simulink model "log2_fixed_point"  (R2018b)
settings: Solver=FixedStepDiscrete  StartTime=0.0  StopTime=1e6  RelTol=1e-3  EnableMultiTasking=on
InitFcn:
  | set_log2_fixed_point_params
undefined symbols (not defined in the file or in its folder): log2_fixed_point
libraries: hdlsllib x22, simulink x8
settings Model: FPTRunName=FPA_Reference  Creator=minimales  LastModifiedBy=ekorotkyi
settings OptimizationCC: BlockReduction=off  ConditionallyExecuteInputs=off  DefaultParameterBehavior=Inlined  LifeSpan=inf
settings DebuggingCC: AlgebraicLoopMsg=error  SingleTaskRateTransMsg=error  SFUnexpectedBacktrackingDiag=warning  SFNoUnconditionalDefaultTransitionDiag=warning  SFExecutionAtInitializationDiag=none
settings HardwareCC: ProdBitPerPointer=32  ProdBitPerSizeT=32  ProdBitPerPtrDiffT=32  ProdLargestAtomicFloat=None  ProdIntDivRoundTo=Undefined  ProdEndianess=Unspecified  ProdWordSize=32  ProdHWDeviceType=ASIC/FPGA->ASIC/FPGA  ProdEqTarget=off
settings SFSimCC: SimUseLocalCustomCode=off
settings RTWCC: RTWUseLocalCustomCode=off
settings CodeAppCC: StateflowObjectComments=on
settings GRTTargetCC: TargetLangStandard=C89/C90 (ANSI)  GeneratePreprocessorConditionals=Disable all
settings ConfigComp: CovScope=Subsystem  CovPath=SIGNAL_PROCESSING_DF  CovMetricSettings=w  CovHTMLOptions=-sRT=1 -sVT=0 -aTS=1 -bRG=1 -bTC=1 -hTR=0 -nFC=0 -nFD=1 -scm=1 -bcm=1 -xEv=0 -xEM=0  CovHtmlReporting=on  CovSaveCumulativeToWorkspaceVar=on  CovSaveSingleToWorkspaceVar=on  CovExternalEMLEnable=off  CovSFcnEnable=off

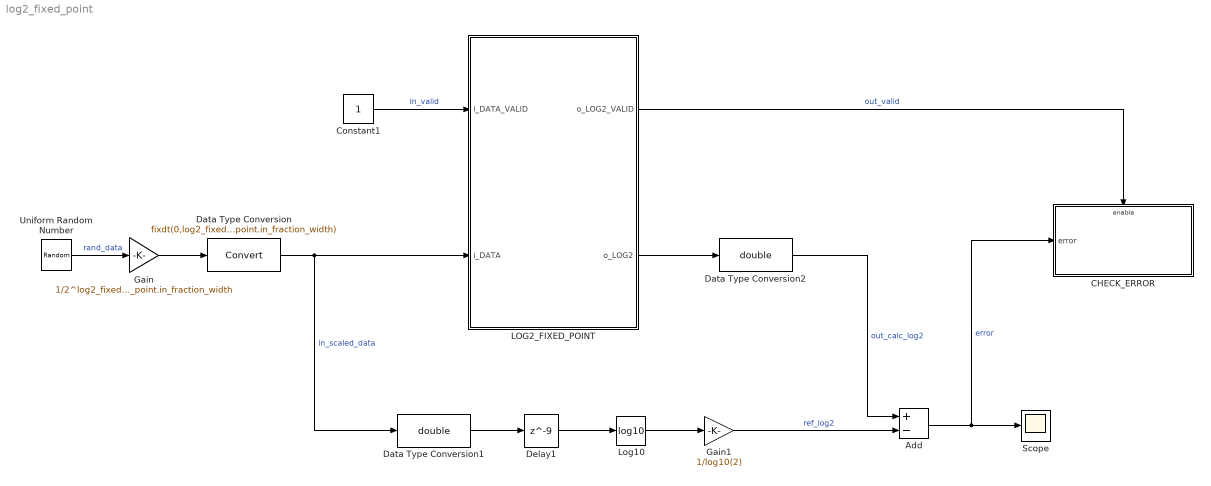
== system log2_fixed_point ==
  Add : Sum  Inputs=+-
  CHECK_ERROR : Subsystem
  Constant1 : Constant  OutDataTypeStr=boolean  SampleTime=1
  Data Type Conversion : DataTypeConversion  OutDataTypeStr=fixdt(0,log2_fixed_point.in_word_width,log2_fixed_point.in_fraction_width)
  Data Type Conversion1 : DataTypeConversion  OutDataTypeStr=double
  Data Type Conversion2 : DataTypeConversion  OutDataTypeStr=double
  Delay1 : Delay  DelayLength=9  InitialCondition=0
  Gain : Gain  Gain=1/2^log2_fixed_point.in_fraction_width
  Gain1 : Gain  Gain=1/log10(2)
  LOG2_FIXED_POINT : Subsystem
  Log10 : Math  Operator=log10  SaturateOnIntegerOverflow=on
  Scope : Scope
  Uniform Random Number : UniformRandomNumber  Minimum=2^(log2_fixed_point.in_word_width-1)  Maximum=2^log2_fixed_point.in_word_width-1  SampleTime=1
  wires:
  LOG2_FIXED_POINT/1(o_LOG2_VALID) -> CHECK_ERROR/Enable  "out_valid"
  LOG2_FIXED_POINT/2(o_LOG2) -> Data Type Conversion2/1
  Constant1/1 -> LOG2_FIXED_POINT/1(i_DATA_VALID)  "in_valid"
  Data Type Conversion/1 -> LOG2_FIXED_POINT/2(i_DATA), Data Type Conversion1/1  "in_scaled_data"
  Log10/1 -> Gain1/1
  Add/1 -> CHECK_ERROR/1(error), Scope/1  "error"
  Gain/1 -> Data Type Conversion/1
  Data Type Conversion2/1 -> Add/1  "out_calc_log2"
  Gain1/1 -> Add/2  "ref_log2"
  Delay1/1 -> Log10/1
  Uniform Random Number/1 -> Gain/1  "rand_data"
  Data Type Conversion1/1 -> Delay1/1

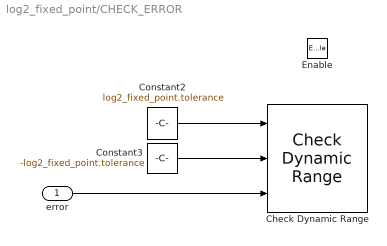
== system log2_fixed_point/CHECK_ERROR ==
  error : Inport
  Enable : EnablePort
  Check Dynamic Range : simulink/Model Verification/Check  Dynamic Range  Description=min < u < max  enabled=on  stopWhenAssertionFail=on  export=off  icon=graphic
      settings: SourceProductName=Simulink  SourceProductBaseCode=SL
  Constant2 : Constant  Value=log2_fixed_point.tolerance  OutDataTypeStr=double  SampleTime=1
  Constant3 : Constant  Value=-log2_fixed_point.tolerance  OutDataTypeStr=double  SampleTime=1
  wires:
  Constant3/1 -> Check Dynamic Range/2
  Constant2/1 -> Check Dynamic Range/1
  error/1 -> Check Dynamic Range/3

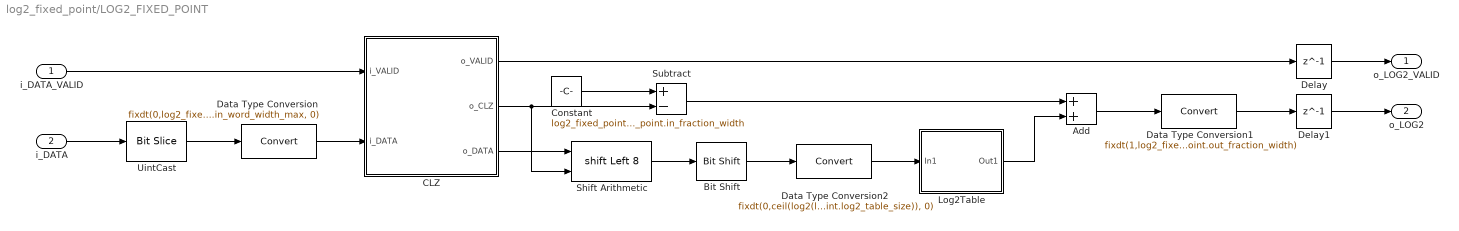
== system log2_fixed_point/LOG2_FIXED_POINT ==
  i_DATA_VALID : Inport  OutDataTypeStr=boolean
  i_DATA : Inport  Port=2  OutDataTypeStr=fixdt(0,log2_fixed_point.in_word_width,log2_fixed_point.in_fraction_width)
  Add : Sum
  Bit Shift : hdlsllib/Logic and Bit Operations/Bit Shift  mode=Shift Right Logical  N=log2_fixed_point.in_word_width_max- (ceil(log2(log2_fixed_point.log2_table_size))+1)
      settings: SourceProductName=HDL Coder  SourceProductBaseCode=HD
  CLZ : Subsystem
  Constant : Constant  Value=log2_fixed_point.in_word_width_max - 1 - log2_fixed_point.in_fraction_width  OutDataTypeStr=fixdt(0,ceil(log2(log2_fixed_point.in_word_width_max)) + 1,0)  SampleTime=1
  Data Type Conversion : DataTypeConversion  OutDataTypeStr=fixdt(0,log2_fixed_point.in_word_width_max, 0)
  Data Type Conversion1 : DataTypeConversion  OutDataTypeStr=fixdt(1,log2_fixed_point.out_word_width,log2_fixed_point.out_fraction_width)
  Data Type Conversion2 : DataTypeConversion  OutDataTypeStr=fixdt(0,ceil(log2(log2_fixed_point.log2_table_size)), 0)
  Delay : Delay  DelayLength=1  InitialCondition=0
  Delay1 : Delay  DelayLength=1  InitialCondition=0
  Log2Table : Subsystem
  Shift Arithmetic : ArithShift  BitShiftNumberSource=Input port  BitShiftNumber=8  BitShiftDirection=Left
      settings: InputPortMap=u0,p1
  Subtract : Sum  Inputs=+-
  UintCast : hdlsllib/Logic and Bit Operations/Bit Slice  lidx=log2_fixed_point.in_word_width-1  ridx=0
  o_LOG2_VALID : Outport
  o_LOG2 : Outport  Port=2
  wires:
  i_DATA_VALID/1 -> CLZ/1(i_VALID)
  i_DATA/1 -> UintCast/1
  CLZ/1(o_VALID) -> Delay/1
  CLZ/2(o_CLZ) -> Shift Arithmetic/2, Subtract/2
  Data Type Conversion/1 -> CLZ/2(i_DATA)
  UintCast/1 -> Data Type Conversion/1
  Constant/1 -> Subtract/1
  Subtract/1 -> Add/1
  CLZ/3(o_DATA) -> Shift Arithmetic/1
  Shift Arithmetic/1 -> Bit Shift/1
  Bit Shift/1 -> Data Type Conversion2/1
  Add/1 -> Data Type Conversion1/1
  Data Type Conversion1/1 -> Delay1/1
  Data Type Conversion2/1 -> Log2Table/1(In1)
  Log2Table/1(Out1) -> Add/2
  Delay/1 -> o_LOG2_VALID/1
  Delay1/1 -> o_LOG2/1

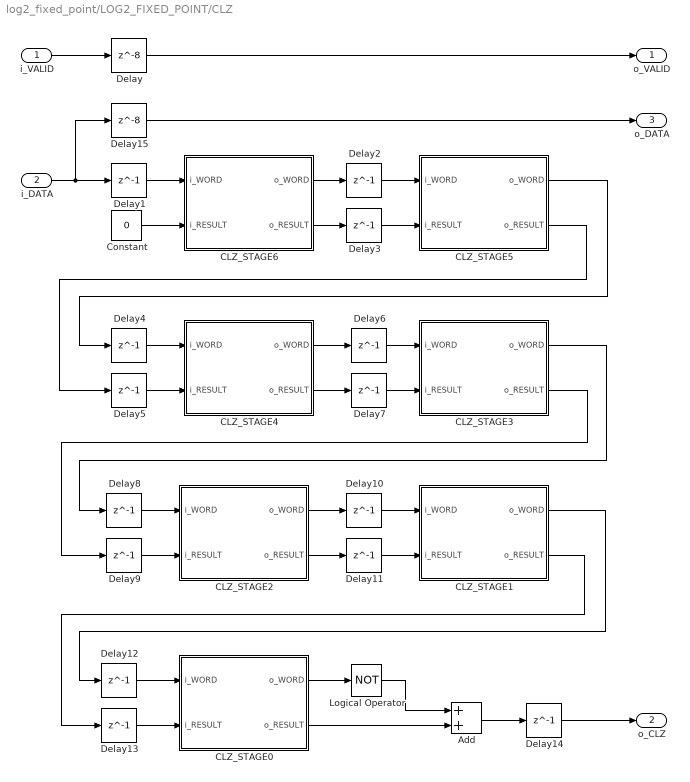
== system log2_fixed_point/LOG2_FIXED_POINT/CLZ ==
  i_VALID : Inport
  i_DATA : Inport  Port=2
  Add : Sum  OutDataTypeStr=fixdt(0,ceil(log2(log2_fixed_point.in_word_width_max)) + 1,0)
  CLZ_STAGE0 : Subsystem
  CLZ_STAGE1 : Subsystem
  CLZ_STAGE2 : Subsystem
  CLZ_STAGE3 : Subsystem
  CLZ_STAGE4 : Subsystem
  CLZ_STAGE5 : Subsystem
  CLZ_STAGE6 : Subsystem
  Constant : Constant  Value=0  OutDataTypeStr=fixdt(0,ceil(log2(log2_fixed_point.in_word_width_max)) + 1,0)  SampleTime=1
  Delay : Delay  DelayLength=8  InitialCondition=0
  Delay{1..14} (14 alike) : Delay  DelayLength=1  InitialCondition=0
  Delay15 : Delay  DelayLength=8  InitialCondition=0
  Logical Operator : Logic  Operator=NOT  AllPortsSameDT=off  OutDataTypeStr=boolean
  o_VALID : Outport
  o_CLZ : Outport  Port=2
  o_DATA : Outport  Port=3
  wires:
  Delay/1 -> o_VALID/1
  i_VALID/1 -> Delay/1
  i_DATA/1 -> Delay15/1, Delay1/1
  Delay1/1 -> CLZ_STAGE6/1(i_WORD)
  Constant/1 -> CLZ_STAGE6/2(i_RESULT)
  CLZ_STAGE6/1(o_WORD) -> Delay2/1
  CLZ_STAGE6/2(o_RESULT) -> Delay3/1
  Delay2/1 -> CLZ_STAGE5/1(i_WORD)
  Delay3/1 -> CLZ_STAGE5/2(i_RESULT)
  Delay4/1 -> CLZ_STAGE4/1(i_WORD)
  Delay5/1 -> CLZ_STAGE4/2(i_RESULT)
  Delay7/1 -> CLZ_STAGE3/2(i_RESULT)
  Delay6/1 -> CLZ_STAGE3/1(i_WORD)
  Delay8/1 -> CLZ_STAGE2/1(i_WORD)
  Delay11/1 -> CLZ_STAGE1/2(i_RESULT)
  Delay9/1 -> CLZ_STAGE2/2(i_RESULT)
  Delay10/1 -> CLZ_STAGE1/1(i_WORD)
  CLZ_STAGE2/1(o_WORD) -> Delay10/1
  CLZ_STAGE2/2(o_RESULT) -> Delay11/1
  Delay13/1 -> CLZ_STAGE0/2(i_RESULT)
  Delay12/1 -> CLZ_STAGE0/1(i_WORD)
  Delay14/1 -> o_CLZ/1
  CLZ_STAGE0/2(o_RESULT) -> Add/2
  CLZ_STAGE0/1(o_WORD) -> Logical Operator/1
  Add/1 -> Delay14/1
  Logical Operator/1 -> Add/1
  CLZ_STAGE5/1(o_WORD) -> Delay4/1
  CLZ_STAGE5/2(o_RESULT) -> Delay5/1
  CLZ_STAGE4/1(o_WORD) -> Delay6/1
  CLZ_STAGE4/2(o_RESULT) -> Delay7/1
  CLZ_STAGE3/1(o_WORD) -> Delay8/1
  CLZ_STAGE3/2(o_RESULT) -> Delay9/1
  CLZ_STAGE1/1(o_WORD) -> Delay12/1
  CLZ_STAGE1/2(o_RESULT) -> Delay13/1
  Delay15/1 -> o_DATA/1

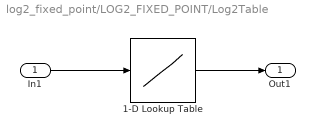
== system log2_fixed_point/LOG2_FIXED_POINT/Log2Table ==
  In1 : Inport
  1-D Lookup Table : Lookup_n-D  NumberOfTableDimensions=1  LookupTableObject=''  BreakpointsForDimension1=[0:log2_fixed_point.log2_table_size-1]  BreakpointsForDimension1FirstPoint=10  BreakpointsForDimension2FirstPoint=10  BreakpointsForDimension1Spacing=12  BreakpointsForDimension2Spacing=12  IndexSearchMethod=Evenly spaced points  Table=log2_fixed_point.log2_table  TableDataTypeStr=Inherit: Inherit from 'Table data'  InterpMethod=Flat  DiagnosticForOutOfRangeInput=Error  InternalRulePriority=Speed  OutDataTypeStr=Inherit: Inherit from 'Table data'  RndMeth=Simplest  InputSameDT=on
  Out1 : Outport
  wires:
  In1/1 -> 1-D Lookup Table/1
  1-D Lookup Table/1 -> Out1/1

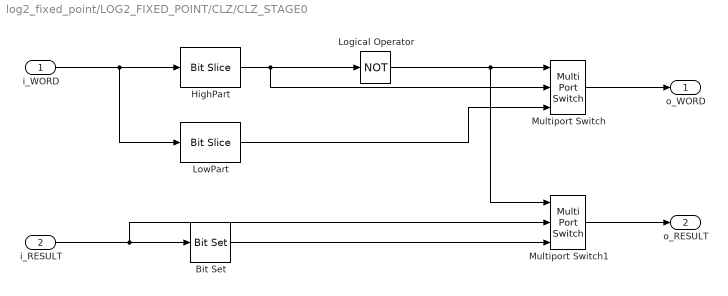
== system log2_fixed_point/LOG2_FIXED_POINT/CLZ/CLZ_STAGE0 ==
  i_WORD : Inport
  i_RESULT : Inport  Port=2
  Bit Set : simulink/Logic and Bit Operations/Bit Set  iBit=0
      settings: SourceProductName=Simulink  SourceProductBaseCode=SL
  HighPart : hdlsllib/Logic and Bit Operations/Bit Slice  lidx=1  ridx=1
  Logical Operator : Logic  Operator=NOT  AllPortsSameDT=off  OutDataTypeStr=boolean
  LowPart : hdlsllib/Logic and Bit Operations/Bit Slice  lidx=0  ridx=0
  Multiport Switch : MultiPortSwitch  DataPortOrder=Zero-based contiguous  Inputs=2  zeroidx=on
  Multiport Switch1 : MultiPortSwitch  DataPortOrder=Zero-based contiguous  Inputs=2  zeroidx=on
  o_WORD : Outport
  o_RESULT : Outport  Port=2
  wires:
  i_RESULT/1 -> Multiport Switch1/2, Bit Set/1
  Multiport Switch/1 -> o_WORD/1
  i_WORD/1 -> LowPart/1, HighPart/1
  Multiport Switch1/1 -> o_RESULT/1
  Logical Operator/1 -> Multiport Switch/1, Multiport Switch1/1
  Bit Set/1 -> Multiport Switch1/3
  HighPart/1 -> Logical Operator/1, Multiport Switch/2
  LowPart/1 -> Multiport Switch/3

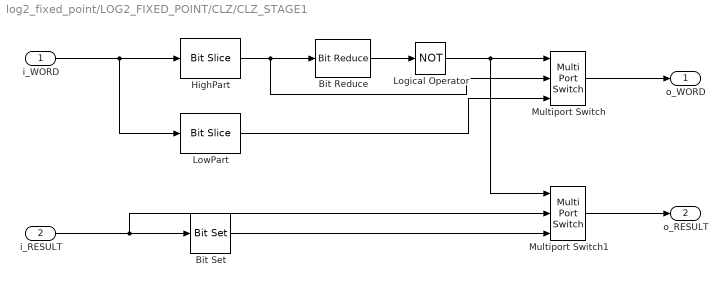
== system log2_fixed_point/LOG2_FIXED_POINT/CLZ/CLZ_STAGE1 ==
  i_WORD : Inport
  i_RESULT : Inport  Port=2
  Bit Reduce : hdlsllib/Logic and Bit Operations/Bit Reduce  mode=OR
      settings: SourceProductName=HDL Coder  SourceProductBaseCode=HD
  Bit Set : simulink/Logic and Bit Operations/Bit Set  iBit=1
      settings: SourceProductName=Simulink  SourceProductBaseCode=SL
  HighPart : hdlsllib/Logic and Bit Operations/Bit Slice  lidx=log2_fixed_point.in_word_width_max/32-1  ridx=log2_fixed_point.in_word_width_max/64
  Logical Operator : Logic  Operator=NOT  AllPortsSameDT=off  OutDataTypeStr=boolean
  LowPart : hdlsllib/Logic and Bit Operations/Bit Slice  lidx=log2_fixed_point.in_word_width_max/64-1  ridx=0
  Multiport Switch : MultiPortSwitch  DataPortOrder=Zero-based contiguous  Inputs=2  zeroidx=on
  Multiport Switch1 : MultiPortSwitch  DataPortOrder=Zero-based contiguous  Inputs=2  zeroidx=on
  o_WORD : Outport
  o_RESULT : Outport  Port=2
  wires:
  i_RESULT/1 -> Multiport Switch1/2, Bit Set/1
  Multiport Switch/1 -> o_WORD/1
  i_WORD/1 -> LowPart/1, HighPart/1
  Multiport Switch1/1 -> o_RESULT/1
  HighPart/1 -> Bit Reduce/1, Multiport Switch/2
  Logical Operator/1 -> Multiport Switch/1, Multiport Switch1/1
  Bit Set/1 -> Multiport Switch1/3
  Bit Reduce/1 -> Logical Operator/1
  LowPart/1 -> Multiport Switch/3

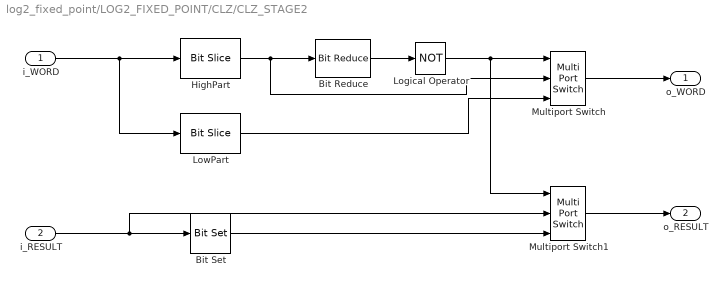
== system log2_fixed_point/LOG2_FIXED_POINT/CLZ/CLZ_STAGE2 ==
  i_WORD : Inport
  i_RESULT : Inport  Port=2
  Bit Reduce : hdlsllib/Logic and Bit Operations/Bit Reduce  mode=OR
      settings: SourceProductName=HDL Coder  SourceProductBaseCode=HD
  Bit Set : simulink/Logic and Bit Operations/Bit Set  iBit=2
      settings: SourceProductName=Simulink  SourceProductBaseCode=SL
  HighPart : hdlsllib/Logic and Bit Operations/Bit Slice  lidx=log2_fixed_point.in_word_width_max/16-1  ridx=log2_fixed_point.in_word_width_max/32
  Logical Operator : Logic  Operator=NOT  AllPortsSameDT=off  OutDataTypeStr=boolean
  LowPart : hdlsllib/Logic and Bit Operations/Bit Slice  lidx=log2_fixed_point.in_word_width_max/32-1  ridx=0
  Multiport Switch : MultiPortSwitch  DataPortOrder=Zero-based contiguous  Inputs=2  zeroidx=on
  Multiport Switch1 : MultiPortSwitch  DataPortOrder=Zero-based contiguous  Inputs=2  zeroidx=on
  o_WORD : Outport
  o_RESULT : Outport  Port=2
  wires:
  i_RESULT/1 -> Multiport Switch1/2, Bit Set/1
  Multiport Switch/1 -> o_WORD/1
  i_WORD/1 -> LowPart/1, HighPart/1
  Multiport Switch1/1 -> o_RESULT/1
  HighPart/1 -> Bit Reduce/1, Multiport Switch/2
  Logical Operator/1 -> Multiport Switch/1, Multiport Switch1/1
  Bit Set/1 -> Multiport Switch1/3
  Bit Reduce/1 -> Logical Operator/1
  LowPart/1 -> Multiport Switch/3

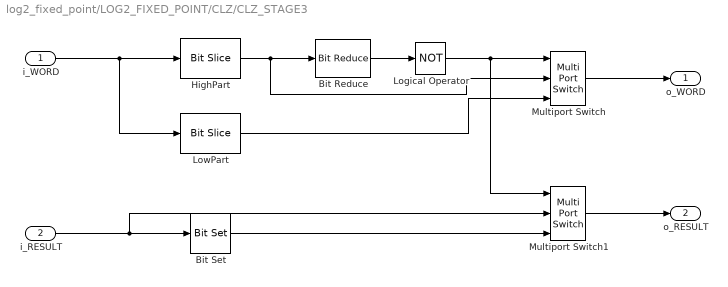
== system log2_fixed_point/LOG2_FIXED_POINT/CLZ/CLZ_STAGE3 ==
  i_WORD : Inport
  i_RESULT : Inport  Port=2
  Bit Reduce : hdlsllib/Logic and Bit Operations/Bit Reduce  mode=OR
      settings: SourceProductName=HDL Coder  SourceProductBaseCode=HD
  Bit Set : simulink/Logic and Bit Operations/Bit Set  iBit=3
      settings: SourceProductName=Simulink  SourceProductBaseCode=SL
  HighPart : hdlsllib/Logic and Bit Operations/Bit Slice  lidx=log2_fixed_point.in_word_width_max/8-1  ridx=log2_fixed_point.in_word_width_max/16
  Logical Operator : Logic  Operator=NOT  AllPortsSameDT=off  OutDataTypeStr=boolean
  LowPart : hdlsllib/Logic and Bit Operations/Bit Slice  lidx=log2_fixed_point.in_word_width_max/16-1  ridx=0
  Multiport Switch : MultiPortSwitch  DataPortOrder=Zero-based contiguous  Inputs=2  zeroidx=on
  Multiport Switch1 : MultiPortSwitch  DataPortOrder=Zero-based contiguous  Inputs=2  zeroidx=on
  o_WORD : Outport
  o_RESULT : Outport  Port=2
  wires:
  i_RESULT/1 -> Multiport Switch1/2, Bit Set/1
  Multiport Switch/1 -> o_WORD/1
  i_WORD/1 -> LowPart/1, HighPart/1
  Multiport Switch1/1 -> o_RESULT/1
  HighPart/1 -> Bit Reduce/1, Multiport Switch/2
  Logical Operator/1 -> Multiport Switch/1, Multiport Switch1/1
  Bit Set/1 -> Multiport Switch1/3
  Bit Reduce/1 -> Logical Operator/1
  LowPart/1 -> Multiport Switch/3

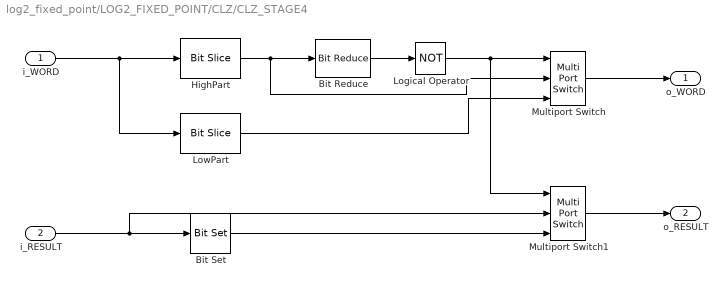
== system log2_fixed_point/LOG2_FIXED_POINT/CLZ/CLZ_STAGE4 ==
  i_WORD : Inport
  i_RESULT : Inport  Port=2
  Bit Reduce : hdlsllib/Logic and Bit Operations/Bit Reduce  mode=OR
      settings: SourceProductName=HDL Coder  SourceProductBaseCode=HD
  Bit Set : simulink/Logic and Bit Operations/Bit Set  iBit=4
      settings: SourceProductName=Simulink  SourceProductBaseCode=SL
  HighPart : hdlsllib/Logic and Bit Operations/Bit Slice  lidx=log2_fixed_point.in_word_width_max/4-1  ridx=log2_fixed_point.in_word_width_max/8
  Logical Operator : Logic  Operator=NOT  AllPortsSameDT=off  OutDataTypeStr=boolean
  LowPart : hdlsllib/Logic and Bit Operations/Bit Slice  lidx=log2_fixed_point.in_word_width_max/8-1  ridx=0
  Multiport Switch : MultiPortSwitch  DataPortOrder=Zero-based contiguous  Inputs=2  zeroidx=on
  Multiport Switch1 : MultiPortSwitch  DataPortOrder=Zero-based contiguous  Inputs=2  zeroidx=on
  o_WORD : Outport
  o_RESULT : Outport  Port=2
  wires:
  i_RESULT/1 -> Multiport Switch1/2, Bit Set/1
  Multiport Switch/1 -> o_WORD/1
  i_WORD/1 -> LowPart/1, HighPart/1
  Multiport Switch1/1 -> o_RESULT/1
  HighPart/1 -> Bit Reduce/1, Multiport Switch/2
  Logical Operator/1 -> Multiport Switch/1, Multiport Switch1/1
  Bit Set/1 -> Multiport Switch1/3
  Bit Reduce/1 -> Logical Operator/1
  LowPart/1 -> Multiport Switch/3

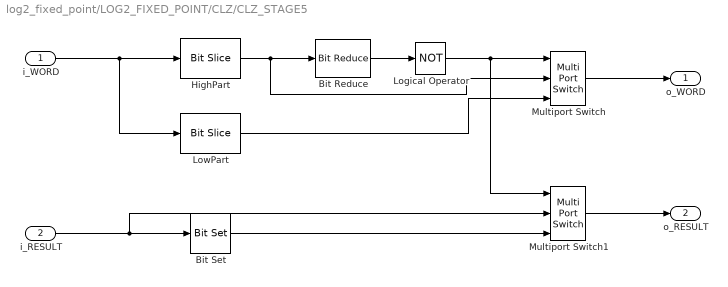
== system log2_fixed_point/LOG2_FIXED_POINT/CLZ/CLZ_STAGE5 ==
  i_WORD : Inport
  i_RESULT : Inport  Port=2
  Bit Reduce : hdlsllib/Logic and Bit Operations/Bit Reduce  mode=OR
      settings: SourceProductName=HDL Coder  SourceProductBaseCode=HD
  Bit Set : simulink/Logic and Bit Operations/Bit Set  iBit=5
      settings: SourceProductName=Simulink  SourceProductBaseCode=SL
  HighPart : hdlsllib/Logic and Bit Operations/Bit Slice  lidx=log2_fixed_point.in_word_width_max/2-1  ridx=log2_fixed_point.in_word_width_max/4
  Logical Operator : Logic  Operator=NOT  AllPortsSameDT=off  OutDataTypeStr=boolean
  LowPart : hdlsllib/Logic and Bit Operations/Bit Slice  lidx=log2_fixed_point.in_word_width_max/4-1  ridx=0
  Multiport Switch : MultiPortSwitch  DataPortOrder=Zero-based contiguous  Inputs=2  zeroidx=on
  Multiport Switch1 : MultiPortSwitch  DataPortOrder=Zero-based contiguous  Inputs=2  zeroidx=on
  o_WORD : Outport
  o_RESULT : Outport  Port=2
  wires:
  i_RESULT/1 -> Multiport Switch1/2, Bit Set/1
  Multiport Switch/1 -> o_WORD/1
  i_WORD/1 -> LowPart/1, HighPart/1
  Multiport Switch1/1 -> o_RESULT/1
  HighPart/1 -> Bit Reduce/1, Multiport Switch/2
  Logical Operator/1 -> Multiport Switch/1, Multiport Switch1/1
  Bit Set/1 -> Multiport Switch1/3
  Bit Reduce/1 -> Logical Operator/1
  LowPart/1 -> Multiport Switch/3

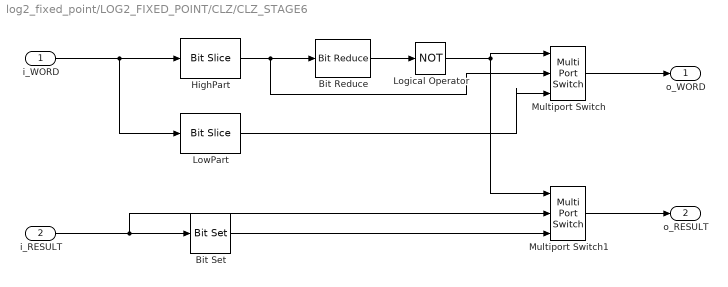
== system log2_fixed_point/LOG2_FIXED_POINT/CLZ/CLZ_STAGE6 ==
  i_WORD : Inport
  i_RESULT : Inport  Port=2
  Bit Reduce : hdlsllib/Logic and Bit Operations/Bit Reduce  mode=OR
      settings: SourceProductName=HDL Coder  SourceProductBaseCode=HD
  Bit Set : simulink/Logic and Bit Operations/Bit Set  iBit=6
      settings: SourceProductName=Simulink  SourceProductBaseCode=SL
  HighPart : hdlsllib/Logic and Bit Operations/Bit Slice  lidx=log2_fixed_point.in_word_width_max-1  ridx=log2_fixed_point.in_word_width_max/2
  Logical Operator : Logic  Operator=NOT  AllPortsSameDT=off  OutDataTypeStr=boolean
  LowPart : hdlsllib/Logic and Bit Operations/Bit Slice  lidx=log2_fixed_point.in_word_width_max/2-1  ridx=0
  Multiport Switch : MultiPortSwitch  DataPortOrder=Zero-based contiguous  Inputs=2  zeroidx=on
  Multiport Switch1 : MultiPortSwitch  DataPortOrder=Zero-based contiguous  Inputs=2  zeroidx=on
  o_WORD : Outport
  o_RESULT : Outport  Port=2
  wires:
  LowPart/1 -> Multiport Switch/3
  i_RESULT/1 -> Multiport Switch1/2, Bit Set/1
  Multiport Switch/1 -> o_WORD/1
  i_WORD/1 -> LowPart/1, HighPart/1
  Multiport Switch1/1 -> o_RESULT/1
  HighPart/1 -> Bit Reduce/1, Multiport Switch/2
  Logical Operator/1 -> Multiport Switch/1, Multiport Switch1/1
  Bit Set/1 -> Multiport Switch1/3
  Bit Reduce/1 -> Logical Operator/1
